simulink model "task4_lin_nonlin_model_MPC_simu"  (R2018a)
settings: Solver=VariableStepAuto  StartTime=0.0  StopTime=100  RelTol=1e-3
values from neighbouring files (symbols this model uses):
  alpha = [alpha1; alpha2]    [OAC_LA_Ass2.m]
  beta = [beta1; beta2]    [OAC_LA_Ass2.m]
  Cd = lin_dsys.C    [OAC_LA_Ass2.m]
  gamma = [gamma1; gamma2]    [OAC_LA_Ass2.m]
  h = evalin('base','h')    [MPC_function.m]    (also in OAC_LA_Ass2.m = [h01; h02])
  h02 = 10.53    [OAC_LA_Ass2.m]
  K = [eye(m),zeros(m,m*(Nc-1))]*inv(H'*Q*H+R)*H'*Q    [OAC_LA_Ass2.m]
  k = [k1; k2]    [OAC_LA_Ass2.m]
  n = size(Ad,1)    [OAC_LA_Ass2.m]
  Ts = 0.5    [OAC_LA_Ass2.m]
  u_eq = evalin('base','u_eq')    [MPC_function.m]    (also in Task1_Funcs.m = [double(S.u1_eq); 0])
  x0_linear = -x_eq + h + ic_liquid_level    [OAC_LA_Ass2.m]
  x0_nonlin = h + ic_liquid_level    [OAC_LA_Ass2.m]
  x_eq = evalin('base','x_eq')    [MPC_function.m]    (also in Task1_Funcs.m = [double(S.x1_eq); x2_eq])
undefined symbols (not defined in the file or in its folder): A, B, F, G
settings Model: Creator=lukastotschnig  LastModifiedBy=miko2

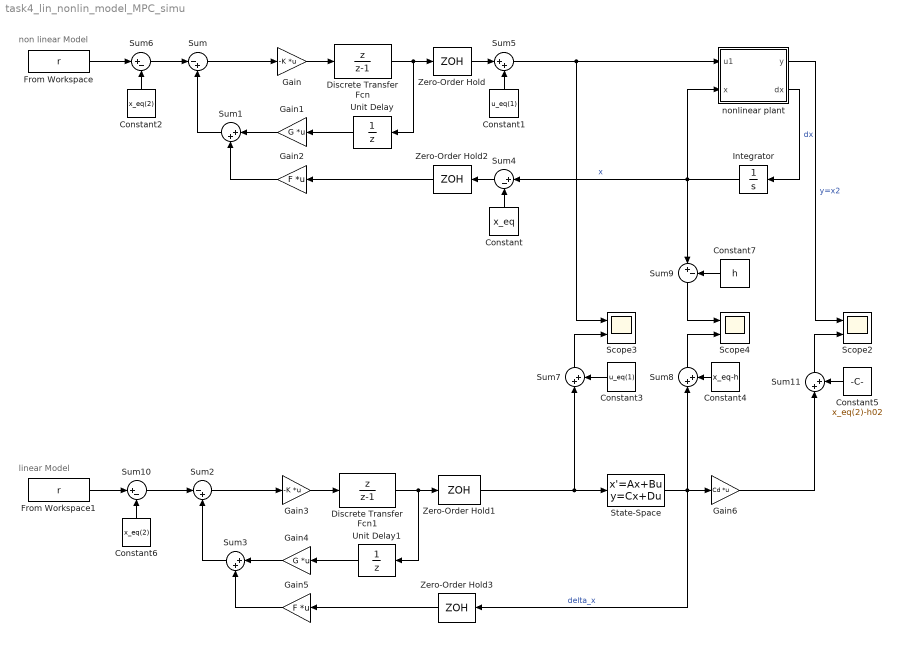
== system task4_lin_nonlin_model_MPC_simu ==
  note: linear Model
  note: non linear Model
  Constant : Constant  Value=x_eq
  Constant1 : Constant  Value=u_eq(1)
  Constant2 : Constant  Value=x_eq(2)
  Constant3 : Constant  Value=u_eq(1)
  Constant4 : Constant  Value=x_eq-h
  Constant5 : Constant  Value=x_eq(2)-h02
  Constant6 : Constant  Value=x_eq(2)
  Constant7 : Constant  Value=h
  Discrete Transfer Fcn : DiscreteTransferFcn  Numerator=[1 0]  Denominator=[1 -1]  SampleTime=Ts
  Discrete Transfer Fcn1 : DiscreteTransferFcn  Numerator=[1 0]  Denominator=[1 -1]  SampleTime=Ts
  From Workspace : FromWorkspace  VariableName=r  SampleTime=0
  From Workspace1 : FromWorkspace  VariableName=r  SampleTime=0
  Gain : Gain  Gain=-K  Multiplication=Matrix(K*u)
  Gain1 : Gain  Gain=G  Multiplication=Matrix(K*u)
  Gain2 : Gain  Gain=F  Multiplication=Matrix(K*u)
  Gain3 : Gain  Gain=-K  Multiplication=Matrix(K*u)
  Gain4 : Gain  Gain=G  Multiplication=Matrix(K*u)
  Gain5 : Gain  Gain=F  Multiplication=Matrix(K*u)
  Gain6 : Gain  Gain=Cd  Multiplication=Matrix(K*u)
  Integrator : Integrator  InitialCondition=x0_nonlin
  Scope2 : Scope  NumInputPorts=2
  Scope3 : Scope  NumInputPorts=2
  Scope4 : Scope  NumInputPorts=2
  State-Space : StateSpace  A=A  B=B  C=eye(n)  D=[0;0]  InitialCondition=x0_linear
  Sum : Sum  Inputs=|-+
  Sum{1,3,5,7..8,11} (6 alike) : Sum  Inputs=|++
  Sum{4,6,9..10} (4 alike) : Sum  Inputs=|+-
  Sum2 : Sum  Inputs=|-+
  Unit Delay : UnitDelay  SampleTime=Ts
  Unit Delay1 : UnitDelay  SampleTime=Ts
  Zero-Order Hold{,1..3} (4 alike) : ZeroOrderHold  SampleTime=Ts
  nonlinear plant : MATLAB Function  TreatAsAtomicUnit=on
  wires:
  nonlinear plant/2(dx) -> Integrator/1  "dx"
  Discrete Transfer Fcn/1 -> Unit Delay/1, Zero-Order Hold/1
  Gain/1 -> Discrete Transfer Fcn/1
  Unit Delay/1 -> Gain1/1
  Sum/1 -> Gain/1
  Gain1/1 -> Sum1/1
  Gain2/1 -> Sum1/2
  Sum1/1 -> Sum/2
  Zero-Order Hold2/1 -> Gain2/1
  Sum4/1 -> Zero-Order Hold2/1
  Constant/1 -> Sum4/2
  Zero-Order Hold/1 -> Sum5/1
  Constant1/1 -> Sum5/2
  From Workspace/1 -> Sum6/1
  Sum6/1 -> Sum/1
  Constant2/1 -> Sum6/2
  Gain4/1 -> Sum3/1
  Sum3/1 -> Sum2/2
  Unit Delay1/1 -> Gain4/1
  Sum10/1 -> Sum2/1
  Gain3/1 -> Discrete Transfer Fcn1/1
  Gain5/1 -> Sum3/2
  Constant6/1 -> Sum10/2
  Zero-Order Hold3/1 -> Gain5/1
  Discrete Transfer Fcn1/1 -> Unit Delay1/1, Zero-Order Hold1/1
  From Workspace1/1 -> Sum10/1
  Sum2/1 -> Gain3/1
  Sum8/1 -> Scope4/2
  Integrator/1 -> Sum9/1, Sum4/1, nonlinear plant/2(x)  "x"
  Gain6/1 -> Sum11/1
  Zero-Order Hold1/1 -> State-Space/1, Sum7/1
  Sum11/1 -> Scope2/2
  Constant5/1 -> Sum11/2
  nonlinear plant/1(y) -> Scope2/1  "y=x2"
  Sum9/1 -> Scope4/1
  State-Space/1 -> Sum8/1, Gain6/1, Zero-Order Hold3/1  "delta_x"
  Constant4/1 -> Sum8/2
  Constant3/1 -> Sum7/2
  Sum7/1 -> Scope3/2
  Constant7/1 -> Sum9/2
  Sum5/1 -> Scope3/1, nonlinear plant/1(u1)

== matlab function task4_lin_nonlin_model_MPC_simu/nonlinear plant ==
  data: y output; dx output; u1 input; x input; k parameter; alpha parameter; beta parameter; gamma parameter; h parameter
function [y, dx]= fcn(u1,x,k,alpha, beta, gamma,h)
    
    % calculate input quantity
    if (beta(1)+gamma(1)*u1) <= 0
        zp1 = 0;
    else
        zp1 = alpha(1) + sqrt( beta(1)+gamma(1)*u1 );
    end
    
    % nonlinear plant description
   dx1 = -k(1)*sqrt(x(1)) + zp1;
   dx2 = -k(2)*sqrt(x(2)) + k(1)*sqrt(x(1));
   
   dx = [dx1; dx2];
   y = x(2)-h(2);

end
